simulink model "PIDFF"  (R2017a)
settings: Solver=VariableStepAuto  StartTime=0.0  StopTime=2000  RelTol=1e-3
libraries: simulink x1
settings Model: Creator=telep  LastModifiedBy=telep

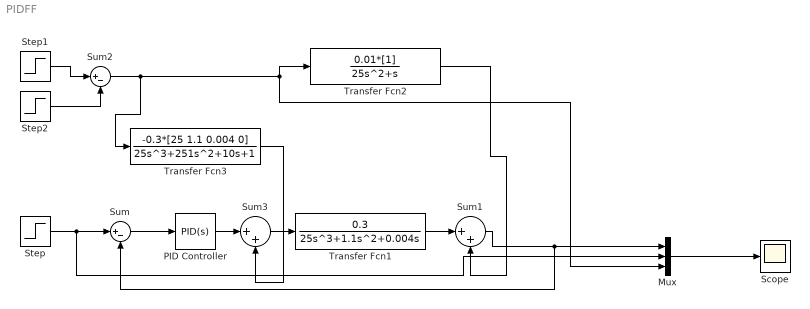
== system PIDFF ==
  Mux : Mux  Inputs=3
  PID Controller : simulink/Continuous/PID Controller  Controller=PID  TimeDomain=Continuous-time  SampleTime=-1  IntegratorMethod=Forward Euler  FilterMethod=Forward Euler  Form=Parallel  UseFilter=on  ControllerParametersSource=internal  P=0.000314838874826811  I=7.49857879656595e-08  D=0.128909794147365  N=3.49324221800777  InitialConditionSource=internal  InitialConditionForIntegrator=0  InitialConditionForFilter=0  ExternalReset=none  LimitOutput=off  UpperSaturationLimit=inf  LowerSaturationLimit=-inf  LinearizeAsGain=on  AntiWindupMode=none  Kb=1  TrackingMode=off  Kt=1  PParamMin=[]  PParamMax=[]  IParamMin=[]  IParamMax=[]  DParamMin=[]  DParamMax=[]  NParamMin=[]  NParamMax=[]  KbParamMin=[]  KbParamMax=[]  KtParamMin=[]  KtParamMax=[]  POutMin=[]  POutMax=[]  IOutMin=[]  IOutMax=[]  DOutMin=[]  DOutMax=[]  NOutMin=[]  NOutMax=[]  KbOutMin=[]  KbOutMax=[]  KtOutMin=[]  KtOutMax=[]  IntegratorOutMin=[]  IntegratorOutMax=[]  FilterOutMin=[]  FilterOutMax=[]  SumOutMin=[]  SumOutMax=[]  SumI1OutMin=[]  SumI1OutMax=[]  SumI2OutMin=[]  SumI2OutMax=[]  SumI3OutMin=[]  SumI3OutMax=[]  SumDOutMin=[]  SumDOutMax=[]  SaturationOutMin=[]  SaturationOutMax=[]  IntegratorContinuousStateAttributes=''  IntegratorStateMustResolveToSignalObject=off  IntegratorRTWStateStorageClass=Auto  FilterContinuousStateAttributes=''  FilterStateMustResolveToSignalObject=off  FilterRTWStateStorageClass=Auto  DifferentiatorICPrevScaledInput=0  DifferentiatorOutMin=[]  DifferentiatorOutMax=[]  InitialConditionSetting=State (most efficient)
  Scope : Scope
  Step : Step  SampleTime=0
  Step1 : Step  Time=1000  SampleTime=0
  Step2 : Step  Time=1100  SampleTime=0
  Sum : Sum  Inputs=|+-
  Sum1 : Sum  Inputs=|++
  Sum2 : Sum  Inputs=|+-
  Sum3 : Sum  Inputs=|++
  Transfer Fcn1 : TransferFcn  Numerator=[0.3]  Denominator=[25 1.1 0.004 0]
  Transfer Fcn2 : TransferFcn  Numerator=0.01*[1]  Denominator=[25 1 0]
  Transfer Fcn3 : TransferFcn  Numerator=-0.3*[25 1.1 0.004 0]  Denominator=[25 251 10 1]
  wires:
  Step/1 -> Sum/1, Mux/2
  Mux/1 -> Scope/1
  Sum/1 -> PID Controller/1
  Transfer Fcn1/1 -> Sum1/1
  Transfer Fcn2/1 -> Sum1/2
  Sum1/1 -> Sum/2, Mux/1
  Sum2/1 -> Transfer Fcn3/1, Transfer Fcn2/1, Mux/3
  Step1/1 -> Sum2/1
  Step2/1 -> Sum2/2
  PID Controller/1 -> Sum3/1
  Sum3/1 -> Transfer Fcn1/1
  Transfer Fcn3/1 -> Sum3/2
